simulink model "sim_backstepping_model"  (R2024a)
settings: Solver=ode4  StartTime=0.0  StopTime=1000.0  FixedStep=0.02  RelTol=1e-3
values from neighbouring files (symbols this model uses):
  D = 0    [linear_model.m]
undefined symbols (not defined in the file or in its folder): c_1, c_2, omega_0, p
settings Model: Creator=marius  LastModifiedBy=marius

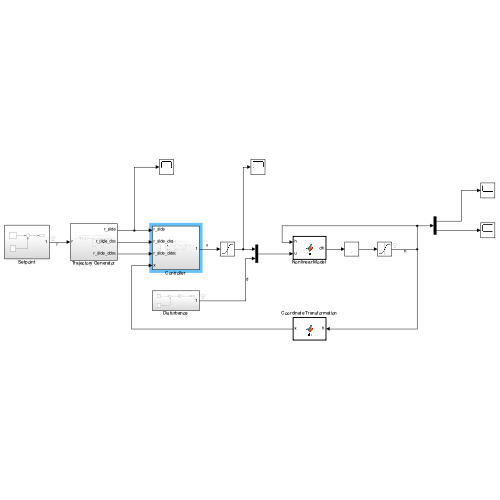
[thumbnail: Simulink's stored preview of the top-level diagram]
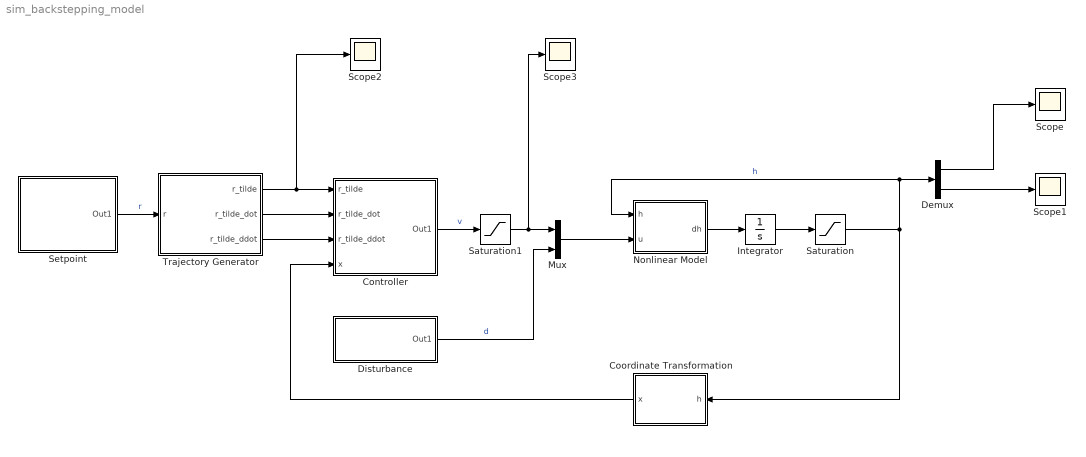
== system sim_backstepping_model ==
  Controller : Subsystem
  Coordinate Transformation : MATLAB Function  TreatAsAtomicUnit=on
  Demux : Demux  Outputs=2
  Disturbance : Subsystem
  Integrator : Integrator  InitialCondition=[p.h1_bar; p.h2_bar]
  Mux : Mux  Inputs=2
  Nonlinear Model : MATLAB Function  TreatAsAtomicUnit=on
  Saturation : Saturate  UpperLimit=0.3  LowerLimit=eps
  Saturation1 : Saturate  UpperLimit=p.v_max  LowerLimit=0
  Scope{,1..3} (4 alike) : Scope
  Setpoint : Subsystem
  Trajectory Generator : Subsystem
  wires:
  Nonlinear Model/1(dh) -> Integrator/1
  Integrator/1 -> Saturation/1
  Mux/1 -> Nonlinear Model/2(u)
  Setpoint/1(Out1) -> Trajectory Generator/1(r)  "r"
  Disturbance/1(Out1) -> Mux/2  "d"
  Demux/1 -> Scope/1
  Demux/2 -> Scope1/1
  Saturation/1 -> Coordinate Transformation/1(h), Nonlinear Model/1(h), Demux/1  "h"
  Controller/1(Out1) -> Saturation1/1  "v"
  Coordinate Transformation/1(x) -> Controller/4(x)
  Trajectory Generator/1(r_tilde) -> Scope2/1, Controller/1(r_tilde)
  Trajectory Generator/2(r_tilde_dot) -> Controller/2(r_tilde_dot)
  Trajectory Generator/3(r_tilde_ddot) -> Controller/3(r_tilde_ddot)
  Saturation1/1 -> Scope3/1, Mux/1

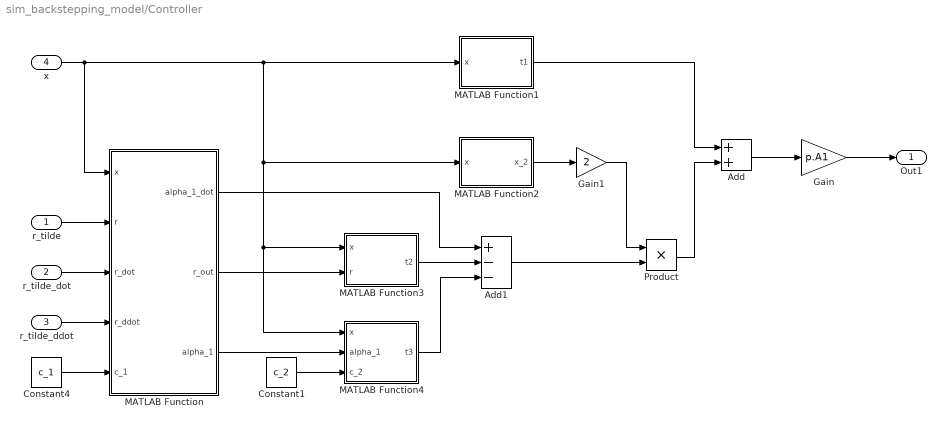
== system sim_backstepping_model/Controller ==
  r_tilde : Inport
  r_tilde_dot : Inport  Port=2
  r_tilde_ddot : Inport  Port=3
  x : Inport  Port=4
  Add : Sum
  Add1 : Sum  Inputs=+--
  Constant1 : Constant  Value=c_2
  Constant4 : Constant  Value=c_1
  Gain : Gain  Gain=p.A1
  Gain1 : Gain  Gain=2
  MATLAB Function : MATLAB Function  TreatAsAtomicUnit=on
  MATLAB Function1 : MATLAB Function  TreatAsAtomicUnit=on
  MATLAB Function2 : MATLAB Function  TreatAsAtomicUnit=on
  MATLAB Function3 : MATLAB Function  TreatAsAtomicUnit=on
  MATLAB Function4 : MATLAB Function  TreatAsAtomicUnit=on
  Product : Product
  Out1 : Outport
  wires:
  MATLAB Function/1(alpha_1_dot) -> Add1/1
  Gain/1 -> Out1/1
  Add/1 -> Gain/1
  MATLAB Function1/1(t1) -> Add/1
  x/1 -> MATLAB Function/1(x), MATLAB Function4/1(x), MATLAB Function3/1(x), MATLAB Function2/1(x), MATLAB Function1/1(x)
  MATLAB Function2/1(x_2) -> Gain1/1
  Product/1 -> Add/2
  Gain1/1 -> Product/1
  Add1/1 -> Product/2
  MATLAB Function3/1(t2) -> Add1/2
  MATLAB Function4/1(t3) -> Add1/3
  Constant1/1 -> MATLAB Function4/3(c_2)
  r_tilde_dot/1 -> MATLAB Function/3(r_dot)
  r_tilde_ddot/1 -> MATLAB Function/4(r_ddot)
  Constant4/1 -> MATLAB Function/5(c_1)
  r_tilde/1 -> MATLAB Function/2(r)
  MATLAB Function/2(r_out) -> MATLAB Function3/2(r)
  MATLAB Function/3(alpha_1) -> MATLAB Function4/2(alpha_1)

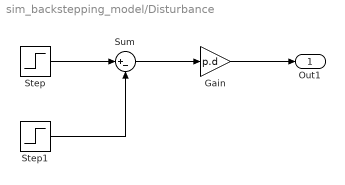
== system sim_backstepping_model/Disturbance ==
  Gain : Gain  Gain=p.d
  Step : Step  Time=p.dt_on  SampleTime=0
  Step1 : Step  Time=p.dt_off  SampleTime=0
  Sum : Sum  Inputs=|+-
  Out1 : Outport
  wires:
  Step/1 -> Sum/1
  Sum/1 -> Gain/1
  Step1/1 -> Sum/2
  Gain/1 -> Out1/1

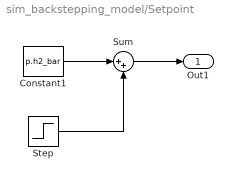
== system sim_backstepping_model/Setpoint ==
  Constant1 : Constant  Value=p.h2_bar
  Step : Step  Time=10  After=0.01  SampleTime=0
  Sum : Sum  Inputs=|++
  Out1 : Outport
  wires:
  Constant1/1 -> Sum/1
  Sum/1 -> Out1/1
  Step/1 -> Sum/2

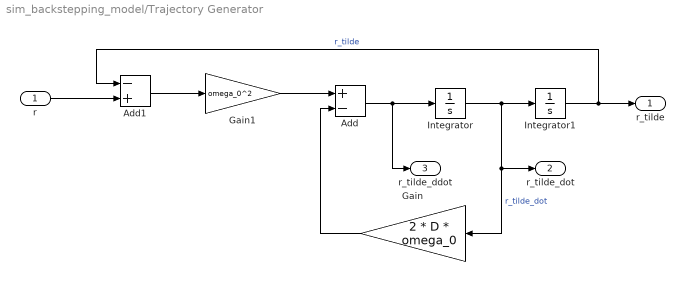
== system sim_backstepping_model/Trajectory Generator ==
  r : Inport
  Add : Sum  Inputs=+-
  Add1 : Sum  Inputs=-+
  Gain : Gain  Gain=2 * D * omega_0
  Gain1 : Gain  Gain=omega_0^2
  Integrator : Integrator
  Integrator1 : Integrator  InitialCondition=p.h2_bar
  r_tilde : Outport
  r_tilde_dot : Outport  Port=2
  r_tilde_ddot : Outport  Port=3
  wires:
  Integrator/1 -> r_tilde_dot/1, Gain/1, Integrator1/1  "r_tilde_dot"
  Add/1 -> r_tilde_ddot/1, Integrator/1
  Integrator1/1 -> Add1/1, r_tilde/1  "r_tilde"
  r/1 -> Add1/2
  Add1/1 -> Gain1/1
  Gain/1 -> Add/2
  Gain1/1 -> Add/1

== matlab function sim_backstepping_model/Coordinate Transformation ==
  data: h input; x output
function x = phi(h)
    x_1 = h(2);
    x_2 = sqrt(h(1));

    x = [x_1; x_2];
end

== matlab function sim_backstepping_model/Nonlinear Model ==
  data: h input; u input; dh output; p parameter
function dh = fcn(h, u, p)
    [dh, y] = nonlinear_model(h, u, p);
end

== matlab function sim_backstepping_model/Controller/MATLAB Function ==
  data: alpha_1_dot output; r_out output; alpha_1 output; x input; r input; r_dot input; r_ddot input; c_1 input; p parameter
function [alpha_1_dot, r_out, alpha_1] = alpha(x, r, r_dot, r_ddot, c_1, p)
    % helper variables
    % dh2 = (1/A2) * (a1*c*x2 - a2*c*sqrt(x1))
    g1 = (p.a1 * p.c) / p.A2;
    f1 = -(p.a2 * p.c * sqrt(x(1))) / p.A2;
    
    % 1. Compute alpha_1
    % z1 = x(1) - r
    alpha_1 = (1/g1) * (r_dot - c_1*(x(1) - r) - f1);
    
    % 2. Derivatives for alpha_1_dot
    % d(f1)/dx1
    df1_dx1 = -(p.a2 * p.c) / (2 * p.A2 * sqrt(x(1)));
    
    dx1 = f1 + g1 * x(2);
    
    % alpha_1_dot = d(alpha1)/dx1 * dx1 + d(alpha1)/dr * dr + d(alpha1)/dr_dot * r_ddot
    term_x1 = (1/g1) * (df1_dx1 - c_1);
    
    alpha_1_dot = term_x1 * dx1 + (1/g1) * (c_1 * r_dot + r_ddot);
    
    r_out = r; % for the layout
end

== matlab function sim_backstepping_model/Controller/MATLAB Function1 ==
  data: x input; t1 output; p parameter
function t1 = term1(x, p)

    t1 = p.k_1 * p.c * x(2);
end

== matlab function sim_backstepping_model/Controller/MATLAB Function2 ==
  data: x input; x_2 output
function x_2 = get_x_2(x)
    x_2 = x(2);
end

== matlab function sim_backstepping_model/Controller/MATLAB Function3 ==
  data: x input; t2 output; r input; p parameter
function t2 = term2(x, r, p)
    t2 = (p.a1/p.A2) * p.c * (x(1) - r);
end

== matlab function sim_backstepping_model/Controller/MATLAB Function4 ==
  data: x input; t3 output; alpha_1 input; c_2 input
function t3 = term3(x, alpha_1, c_2)
    t3 = c_2 * (x(2) - alpha_1);
end
